simulink model "TESTENV_SignalIntegrity"  (R2020a)
settings: Solver=ode1  StartTime=tspan(1)  StopTime=tspan(2)  FixedStep=1/sensorFs.imuUpdateFs  RelTol=1e-3
settings Model: PauseTimes=1  PacingRate=5  Creator=sl  LastModifiedBy=Administrator
settings SolverCC: AutoInsertRateTranBlk=on
settings OptimizationCC: DefaultParameterBehavior=Inlined  EnhancedBackFolding=on  PassReuseOutputArgsAs=Individual arguments  ZeroExternalMemoryAtStartup=off  ZeroInternalMemoryAtStartup=off  MaxStackSize=64  OptimizeBlockOrder=speed  DifferentSizesBufferReuse=on  OptimizationCustomize=off  EfficientTunableParamExpr=on
settings DebuggingCC: MultiTaskCondExecSysMsg=none  ParameterTunabilityLossMsg=error  UnconnectedInputMsg=none  UnconnectedOutputMsg=none  UnconnectedLineMsg=none  BusObjectLabelMismatch=error
settings HardwareCC: ProdBitPerPointer=32  ProdBitPerSizeT=32  ProdBitPerPtrDiffT=32  ProdLargestAtomicInteger=Long  ProdLargestAtomicFloat=Double  ProdWordSize=32  ProdHWDeviceType=ARM Compatible->ARM Cortex
settings ModelReferenceCC: EnableParallelModelReferenceBuilds=on  ParallelModelReferenceMATLABWorkerInit=Load Top Model
settings SFSimCC: MATLABDynamicMemAlloc=off
settings RTWCC: SystemTargetFile=ert.tlc  TemplateMakefile=ert_default_tmf  GenerateReport=on  Toolchain=GNU Tools for ARM Embedded Processors  IncludeHyperlinkInReport=on  LaunchReport=on  GenerateTraceInfo=on  GenerateTraceReport=on  GenerateTraceReportSl=on  GenerateTraceReportSf=on  GenerateTraceReportEml=on
settings CodeAppCC: ForceParamTrailComments=on  IgnoreCustomStorageClasses=off  OperatorAnnotations=on  SimulinkDataObjDesc=on  SFDataObjDesc=on  InsertBlockDesc=on
settings ERTTargetCC: InlinedParameterPlacement=NonHierarchical  ERTCustomFileTemplate=example_file_process.tlc

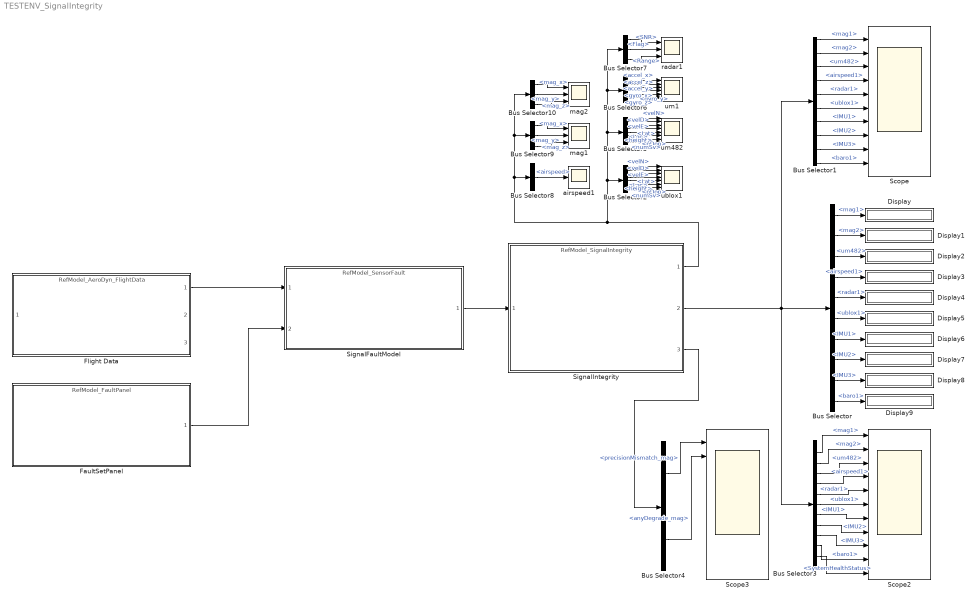
== system TESTENV_SignalIntegrity ==
  Bus Selector : BusSelector  OutputSignals=sensorLostTime.mag1,sensorLostTime.mag2,sensorLostTime.um482,sensorLostTime.airspeed1,sensorLostTime.radar1,sensorLostTime.ublox1,sensorLostTime.IMU1,sensorLostTime.IMU2,sensorLostTime.IMU3,sensorLostTime.baro1
  Bus Selector1 : BusSelector  OutputSignals=sensorLostTime.mag1,sensorLostTime.mag2,sensorLostTime.um482,sensorLostTime.airspeed1,sensorLostTime.radar1,sensorLostTime.ublox1,sensorLostTime.IMU1,sensorLostTime.IMU2,sensorLostTime.IMU3,sensorLostTime.baro1
  Bus Selector10 : BusSelector  OutputSignals=mag2.mag_x,mag2.mag_y,mag2.mag_z
  Bus Selector2 : BusSelector  OutputSignals=ublox1.velN,ublox1.velE,ublox1.velD,ublox1.Lat,ublox1.Lon,ublox1.height,ublox1.pDop,ublox1.numSv
  Bus Selector3 : BusSelector  OutputSignals=SensorStatus.mag1,SensorStatus.mag2,SensorStatus.um482,SensorStatus.airspeed1,SensorStatus.radar1,SensorStatus.ublox1,SensorStatus.IMU1,SensorStatus.IMU2,SensorStatus.IMU3,SensorStatus.baro1,SystemHealthStatus
  Bus Selector4 : BusSelector  OutputSignals=precisionMismatch_mag,anyDegrade_mag
  Bus Selector5 : BusSelector  OutputSignals=um482.velN,um482.velE,um482.velD,um482.Lat,um482.Lon,um482.height,um482.pDop,um482.numSv
  Bus Selector6 : BusSelector  OutputSignals=IMU1.accel_x,IMU1.accel_y,IMU1.accel_z,IMU1.gyro_x,IMU1.gyro_y,IMU1.gyro_z
  Bus Selector7 : BusSelector  OutputSignals=radar1.SNR,radar1.Flag,radar1.Range
  Bus Selector8 : BusSelector  OutputSignals=airspeed1.airspeed
  Bus Selector9 : BusSelector  OutputSignals=mag1.mag_x,mag1.mag_y,mag1.mag_z
  Display{,1..9} (10 alike) : Display
  FaultSetPanel : ModelReference  ModelNameDialog=RefModel_FaultPanel  SimulationMode=Normal  ModelReferenceVersion=1.1481
  Flight Data : ModelReference  DisableCoverage=on  ModelNameDialog=RefModel_AeroDyn_FlightData.slx  SimulationMode=Normal  ModelReferenceVersion=1.1294
  Scope : Scope  NumInputPorts=10
  Scope2 : Scope  NumInputPorts=11
  Scope3 : Scope  NumInputPorts=10
  SignalFaultModel : ModelReference  DisableCoverage=on  ModelNameDialog=RefModel_SensorFault.slx  SimulationMode=Normal  ModelReferenceVersion=1.387
  SignalIntegrity : ModelReference  DisableCoverage=on  ModelNameDialog=RefModel_SignalIntegrity.slx  SimulationMode=Normal  CachedPortDiscreteRates=[0.004;0.4]  ModelReferenceVersion=1.616
  airspeed1 : Scope
  mag1 : Scope  NumInputPorts=3
  mag2 : Scope  NumInputPorts=3
  radar1 : Scope  NumInputPorts=3
  ublox1 : Scope  NumInputPorts=8
  um1 : Scope  NumInputPorts=6
  um482 : Scope  NumInputPorts=8
  wires:
  Bus Selector/1 -> Display/1  "<mag1>"
  Bus Selector/2 -> Display1/1  "<mag2>"
  Bus Selector/3 -> Display2/1  "<um482>"
  Bus Selector/4 -> Display3/1  "<airspeed1>"
  Bus Selector/5 -> Display4/1  "<radar1>"
  Bus Selector/6 -> Display5/1  "<ublox1>"
  Bus Selector/7 -> Display6/1  "<IMU1>"
  Bus Selector/8 -> Display7/1  "<IMU2>"
  Bus Selector/9 -> Display8/1  "<IMU3>"
  Bus Selector/10 -> Display9/1  "<baro1>"
  Bus Selector1/1 -> Scope/1  "<mag1>"
  Bus Selector1/2 -> Scope/2  "<mag2>"
  Bus Selector1/3 -> Scope/3  "<um482>"
  Bus Selector1/4 -> Scope/4  "<airspeed1>"
  Bus Selector1/5 -> Scope/5  "<radar1>"
  Bus Selector1/6 -> Scope/6  "<ublox1>"
  Bus Selector1/7 -> Scope/7  "<IMU1>"
  Bus Selector1/8 -> Scope/8  "<IMU2>"
  Bus Selector1/9 -> Scope/9  "<IMU3>"
  Bus Selector1/10 -> Scope/10  "<baro1>"
  Bus Selector2/1 -> ublox1/1  "<velN>"
  Bus Selector3/10 -> Scope2/10  "<baro1>"
  Bus Selector3/9 -> Scope2/9  "<IMU3>"
  Bus Selector3/8 -> Scope2/8  "<IMU2>"
  Bus Selector3/7 -> Scope2/7  "<IMU1>"
  Bus Selector3/6 -> Scope2/6  "<ublox1>"
  Bus Selector3/5 -> Scope2/5  "<radar1>"
  Bus Selector3/3 -> Scope2/3  "<um482>"
  Bus Selector3/2 -> Scope2/2  "<mag2>"
  Bus Selector3/1 -> Scope2/1  "<mag1>"
  SignalIntegrity/2 -> Bus Selector1/1, Bus Selector3/1, Bus Selector/1
  Bus Selector3/4 -> Scope2/4  "<airspeed1>"
  SignalFaultModel/1 -> SignalIntegrity/1
  Flight Data/1 -> SignalFaultModel/1
  Bus Selector4/1 -> Scope3/1  "<precisionMismatch_mag>"
  Bus Selector4/2 -> Scope3/2  "<anyDegrade_mag>"
  SignalIntegrity/3 -> Bus Selector4/1
  FaultSetPanel/1 -> SignalFaultModel/2
  Bus Selector2/2 -> ublox1/2  "<velE>"
  Bus Selector2/3 -> ublox1/3  "<velD>"
  Bus Selector2/4 -> ublox1/4  "<Lat>"
  Bus Selector2/5 -> ublox1/5  "<Lon>"
  Bus Selector2/6 -> ublox1/6  "<height>"
  Bus Selector2/7 -> ublox1/7  "<pDop>"
  Bus Selector2/8 -> ublox1/8  "<numSv>"
  Bus Selector5/1 -> um482/1  "<velN>"
  Bus Selector5/2 -> um482/2  "<velE>"
  Bus Selector5/3 -> um482/3  "<velD>"
  Bus Selector5/4 -> um482/4  "<Lat>"
  Bus Selector5/5 -> um482/5  "<Lon>"
  Bus Selector5/6 -> um482/6  "<height>"
  Bus Selector5/7 -> um482/7  "<pDop>"
  Bus Selector5/8 -> um482/8  "<numSv>"
  Bus Selector6/1 -> um1/1  "<accel_x>"
  Bus Selector6/2 -> um1/2  "<accel_y>"
  Bus Selector6/3 -> um1/3  "<accel_z>"
  Bus Selector6/4 -> um1/4  "<gyro_x>"
  Bus Selector6/5 -> um1/5  "<gyro_y>"
  Bus Selector6/6 -> um1/6  "<gyro_z>"
  Bus Selector7/2 -> radar1/2  "<Flag>"
  Bus Selector7/1 -> radar1/1  "<SNR>"
  Bus Selector7/3 -> radar1/3  "<Range>"
  SignalIntegrity/1 -> Bus Selector10/1, Bus Selector9/1, Bus Selector8/1, Bus Selector7/1, Bus Selector6/1, Bus Selector5/1, Bus Selector2/1
  Bus Selector8/1 -> airspeed1/1  "<airspeed>"
  Bus Selector9/1 -> mag1/1  "<mag_x>"
  Bus Selector9/2 -> mag1/2  "<mag_y>"
  Bus Selector9/3 -> mag1/3  "<mag_z>"
  Bus Selector10/3 -> mag2/3  "<mag_z>"
  Bus Selector10/2 -> mag2/2  "<mag_y>"
  Bus Selector10/1 -> mag2/1  "<mag_x>"
  Bus Selector3/11 -> Scope2/11  "<SystemHealthStatus>"
